simulink model "Simulink"  (R2023b)
settings: Solver=ode4  StartTime=0.0  StopTime=1  FixedStep=0.0167  RelTol=1e-3
undefined symbols (not defined in the file or in its folder): A, B
settings Model: Creator=vadim  LastModifiedBy=vadim

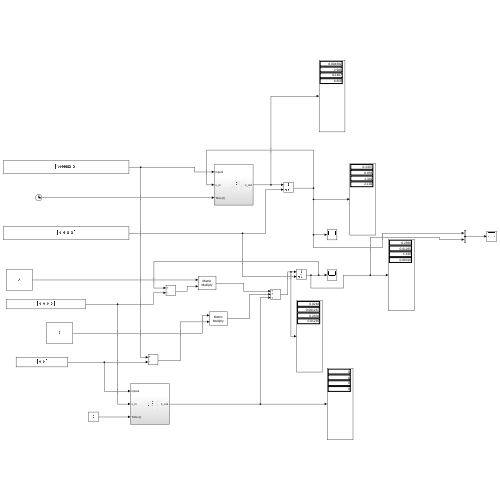
[thumbnail: Simulink's stored preview of the top-level diagram]
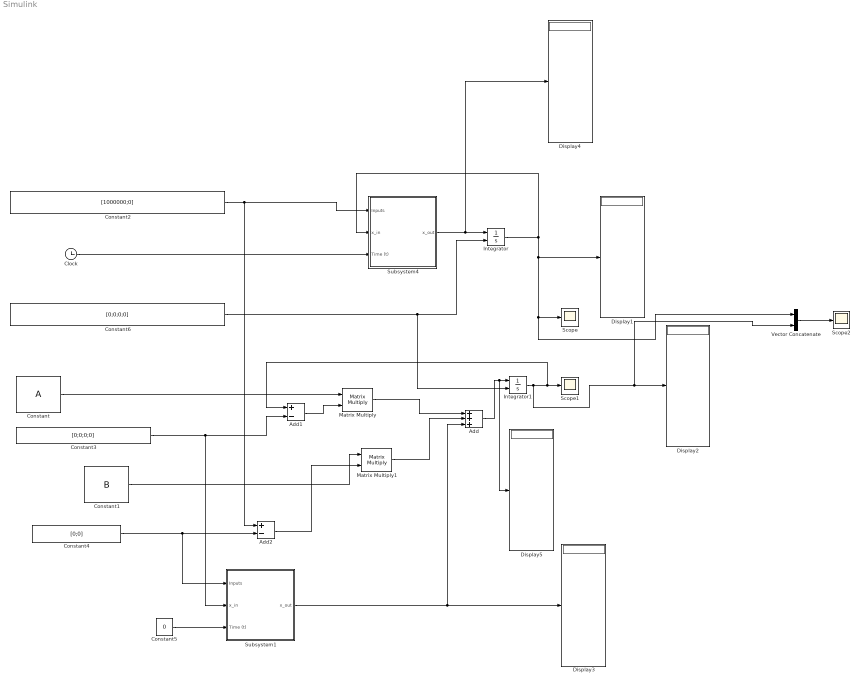
== system Simulink ==
  Add : Sum  Inputs=+++
  Add1 : Sum  Inputs=+-
  Add2 : Sum  Inputs=+-
  Clock : Clock
  Constant : Constant  Value=A
  Constant1 : Constant  Value=B
  Constant2 : Constant  Value=[1000000;0]
  Constant3 : Constant  Value=[0;0;0;0]
  Constant4 : Constant  Value=[0;0]
  Constant5 : Constant  Value=0
  Constant6 : Constant  Value=[0;0;0;0]
  Display{1..5} (5 alike) : Display
  Integrator : Integrator  InitialConditionSource=external
  Integrator1 : Integrator  InitialConditionSource=external
  Matrix Multiply : Product  Multiplication=Matrix(*)
  Matrix Multiply1 : Product  Multiplication=Matrix(*)
  Scope : Scope
  Scope1 : Scope
  Scope2 : Scope
  Subsystem1 : Subsystem
  Subsystem4 : Subsystem
  Vector Concatenate : Concatenate
  wires:
  Constant1/1 -> Matrix Multiply1/1
  Subsystem4/1(x_out) -> Display4/1, Integrator/1
  Clock/1 -> Subsystem4/3(Time (t))
  Matrix Multiply/1 -> Add/1
  Add/1 -> Display5/1, Integrator1/1
  Integrator/1 -> Vector Concatenate/1, Scope/1, Display1/1, Subsystem4/2(x_in)
  Constant2/1 -> Subsystem4/1(Inputs), Add2/1
  Constant6/1 -> Integrator1/2, Integrator/2
  Integrator1/1 -> Vector Concatenate/2, Display2/1, Add1/1, Scope1/1
  Matrix Multiply1/1 -> Add/2
  Constant/1 -> Matrix Multiply/1
  Constant3/1 -> Subsystem1/2(x_in), Add1/2
  Constant4/1 -> Subsystem1/1(Inputs), Add2/2
  Add2/1 -> Matrix Multiply1/2
  Add1/1 -> Matrix Multiply/2
  Constant5/1 -> Subsystem1/3(Time (t))
  Subsystem1/1(x_out) -> Display3/1, Add/3
  Vector Concatenate/1 -> Scope2/1

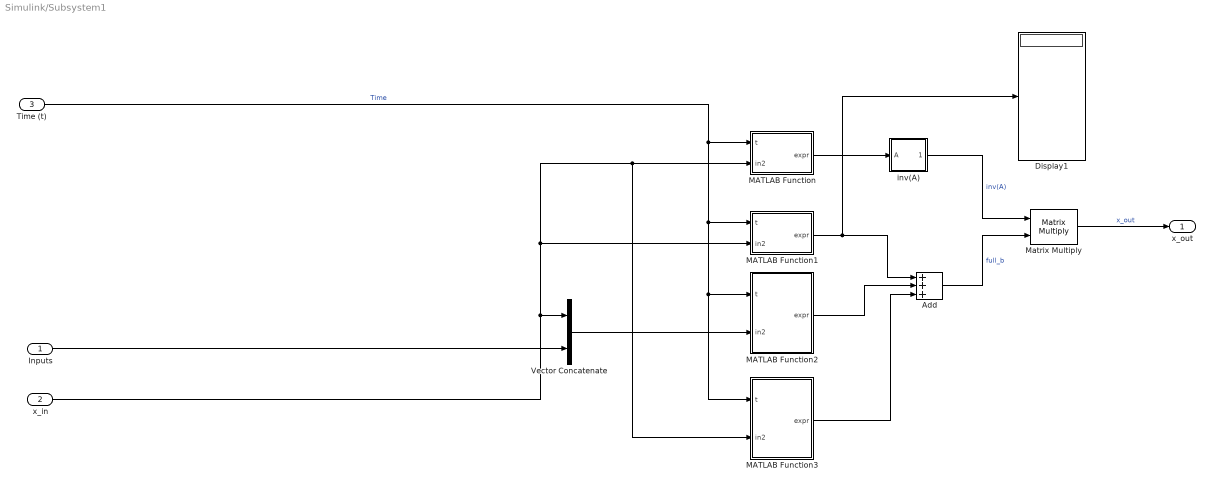
== system Simulink/Subsystem1 ==
  Inputs : Inport
  x_in : Inport  Port=2
  Time (t) : Inport  Port=3
  Add : Sum  Inputs=+++
  Display1 : Display
  MATLAB Function : MATLAB Function  TreatAsAtomicUnit=on
  MATLAB Function1 : MATLAB Function  TreatAsAtomicUnit=on
  MATLAB Function2 : MATLAB Function  TreatAsAtomicUnit=on
  MATLAB Function3 : MATLAB Function  TreatAsAtomicUnit=on
  Matrix Multiply : Product  Multiplication=Matrix(*)
  Vector Concatenate : Concatenate
  inv(A) : Subsystem
  x_out : Outport
  wires:
  MATLAB Function1/1(expr) -> Display1/1, Add/1
  MATLAB Function2/1(expr) -> Add/2
  x_in/1 -> MATLAB Function3/2(in2), MATLAB Function/2(in2), MATLAB Function1/2(in2), Vector Concatenate/1
  inv(A)/1(Out1) -> Matrix Multiply/1  "inv(A)"
  Add/1 -> Matrix Multiply/2  "full_b"
  Matrix Multiply/1 -> x_out/1  "x_out"
  Vector Concatenate/1 -> MATLAB Function2/2(in2)
  Time (t)/1 -> MATLAB Function3/1(t), MATLAB Function2/1(t), MATLAB Function1/1(t), MATLAB Function/1(t)  "Time"
  Inputs/1 -> Vector Concatenate/2
  MATLAB Function/1(expr) -> inv(A)/1(A)
  MATLAB Function3/1(expr) -> Add/3

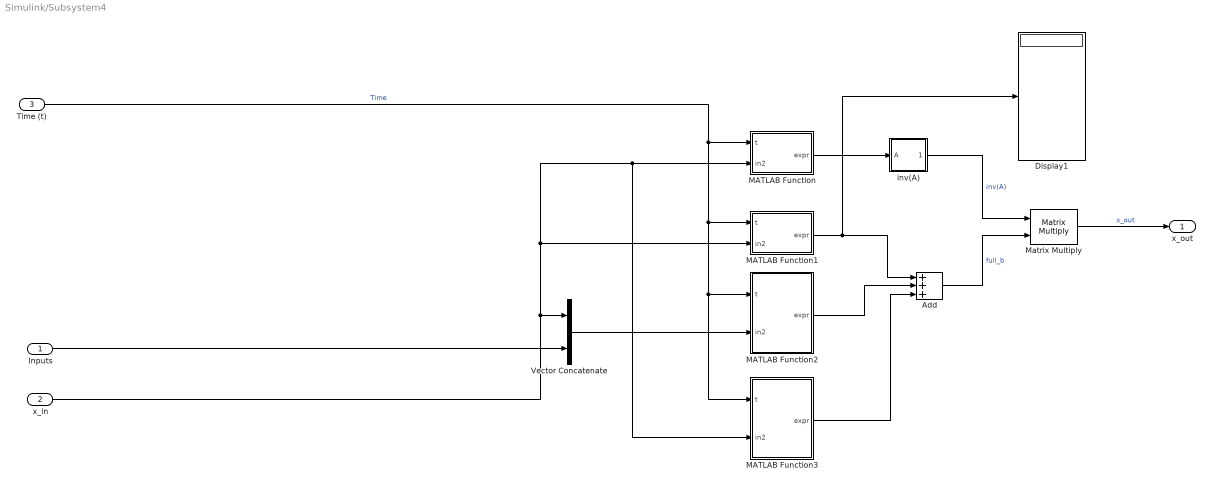
== system Simulink/Subsystem4 ==
  Inputs : Inport
  x_in : Inport  Port=2
  Time (t) : Inport  Port=3
  Add : Sum  Inputs=+++
  Display1 : Display
  MATLAB Function : MATLAB Function  TreatAsAtomicUnit=on
  MATLAB Function1 : MATLAB Function  TreatAsAtomicUnit=on
  MATLAB Function2 : MATLAB Function  TreatAsAtomicUnit=on
  MATLAB Function3 : MATLAB Function  TreatAsAtomicUnit=on
  Matrix Multiply : Product  Multiplication=Matrix(*)
  Vector Concatenate : Concatenate
  inv(A) : Subsystem
  x_out : Outport
  wires:
  MATLAB Function1/1(expr) -> Display1/1, Add/1
  MATLAB Function2/1(expr) -> Add/2
  x_in/1 -> MATLAB Function3/2(in2), MATLAB Function/2(in2), MATLAB Function1/2(in2), Vector Concatenate/1
  inv(A)/1(Out1) -> Matrix Multiply/1  "inv(A)"
  Add/1 -> Matrix Multiply/2  "full_b"
  Matrix Multiply/1 -> x_out/1  "x_out"
  Vector Concatenate/1 -> MATLAB Function2/2(in2)
  Time (t)/1 -> MATLAB Function3/1(t), MATLAB Function2/1(t), MATLAB Function1/1(t), MATLAB Function/1(t)  "Time"
  Inputs/1 -> Vector Concatenate/2
  MATLAB Function/1(expr) -> inv(A)/1(A)
  MATLAB Function3/1(expr) -> Add/3

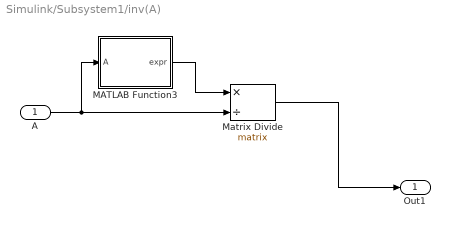
== system Simulink/Subsystem1/inv(A) ==
  A : Inport
  MATLAB Function3 : MATLAB Function  TreatAsAtomicUnit=on
  Matrix Divide : Product  Inputs=*/  Multiplication=Matrix(*)
  Out1 : Outport
  wires:
  MATLAB Function3/1(expr) -> Matrix Divide/1
  A/1 -> Matrix Divide/2, MATLAB Function3/1(A)
  Matrix Divide/1 -> Out1/1

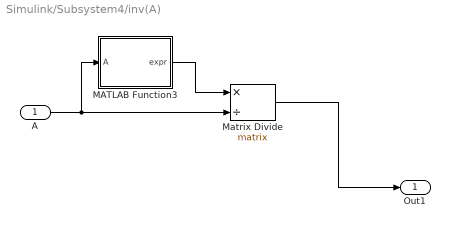
== system Simulink/Subsystem4/inv(A) ==
  A : Inport
  MATLAB Function3 : MATLAB Function  TreatAsAtomicUnit=on
  Matrix Divide : Product  Inputs=*/  Multiplication=Matrix(*)
  Out1 : Outport
  wires:
  MATLAB Function3/1(expr) -> Matrix Divide/1
  A/1 -> Matrix Divide/2, MATLAB Function3/1(A)
  Matrix Divide/1 -> Out1/1

== matlab function Simulink/Subsystem1/MATLAB Function ==
  data: t input; expr output; in2 input
function expr = A(t,in2)
expr = A_uv(t,in2);
end

== matlab function Simulink/Subsystem1/MATLAB Function1 ==
  data: t input; expr output; in2 input
function expr = b(t,in2)

expr = b_uv(t,in2);

end

== matlab function Simulink/Subsystem1/MATLAB Function2 ==
  data: t input; expr output; in2 input
function expr = input_b(t,in2)

expr = input_b_uv(t,in2);

end

== matlab function Simulink/Subsystem1/MATLAB Function3 ==
  data: t input; expr output; in2 input
function expr = v(t,in2)

expr = v_uv(t,in2);

end

== matlab function Simulink/Subsystem1/inv(A)/MATLAB Function3 ==
  data: A input; expr output
function expr = EYE(A)
n = size(A);
expr = eye(n);
end

== matlab function Simulink/Subsystem4/MATLAB Function ==
  data: t input; expr output; in2 input
function expr = A(t,in2)
expr = A_uv(t,in2);
end

== matlab function Simulink/Subsystem4/MATLAB Function1 ==
  data: t input; expr output; in2 input
function expr = b(t,in2)

expr = b_uv(t,in2);

end

== matlab function Simulink/Subsystem4/MATLAB Function2 ==
  data: t input; expr output; in2 input
function expr = input_b(t,in2)

expr = input_b_uv(t,in2);

end

== matlab function Simulink/Subsystem4/inv(A)/MATLAB Function3 ==
  data: A input; expr output
function expr = EYE(A)
n = size(A);
expr = eye(n);
end

== matlab function Simulink/Subsystem4/MATLAB Function3 ==
  data: t input; expr output; in2 input
function expr = v(t,in2)

expr = v_uv(t,in2);

end
